simulink model "vipldws_fixpt"  (R2015b)
settings: Solver=FixedStepDiscrete  StartTime=0.0  StopTime=inf  RelTol=1e-3
model workspace (MATLAB code in the model file):
  | % Image size
  | imgSize = [240 360];
  | 
  | % Number of rows and columns in the image region to process.
  | numRows = floor(imgSize(1)/2);
  | numCols = imgSize(2);
  | 
  | % To handle different video sizes other than [240 360], scaling the Hough
  | % transform rho values by the below factor is required.
  | factor = sqrt(sum(imgSize.^2)) / sqrt(sum([240 360].^2));
  | 
  | %% parameters for the second lane
  | %approximately 35:45 (0-based index: 414:424)
  | startIdxRho_R = floor(factor * 414);
  | NumRhos_R = floor(factor * 11);
  | 
  | %approximately -90:-70 degrees (0-based index: 0:20)
  | startIdxTheta_R = 0;
  | NumThetas_R = 21;
  | neighborhood_R =  [min(7,NumRhos_R), min(7,NumThetas_R)];
  | 
  | %approximately 379:415 (0-based index: 0:35)
  | startIdxRho_L = floor(factor * 379);
  | NumRhos_L = floor(factor * 36);
  | 
  | %approximately 55:85 degrees (0-based index: 145: 175)
  | startIdxTheta_L = 145;
  | NumThetas_L = 21;
  | neighborhood_L =  [min(7,NumRhos_L), min(7,NumThetas_L)];
  | 
  | % Maximum number of lanes to find in the current frame.
  | expLaneNum = 2;
  | 
  | % Maximum number of lanes to store in the tracking repository.
  | maxLaneNum = 20;
  | 
  | % Angular resolution of Hough transform, i.e., the width of a theta bin is
  | % pi/angleNum.
  | angleNum = 180;
  | 
  | % Maximum allowable change of lane distance metric between two frames.
  | trackThreshold = 75;
  | 
  | % Minimum number of frames a lane must be detected to become a valid lane.
  | frameFound = 5;
  | 
  | % Maximum number of frames a lane can be missed without marking it invalid.
  | frameLost = 20;
  | 
  | % Size of the neighborhood around the maxima over which the Hough
  | % transforms values are suppressed. (Used in Find Local Maxima block)
  | neighborhood = [301, 81];
  | 
  | % Distance threshold for lane crossing warning; valid range is (0, 0.5).
  | thrWarn = 0.4;
  | 
  | % Weight (tweaking factor) of the angular difference for calculating the
  | % distance metric between two lanes. It is typically chosen to be close
  | % to the input image rows.
  | distanceMetricWeight = 200;
  | 
  | % Audio track used for lane cross warning.
  | load viprumbling.mat;
values from neighbouring files (symbols this model uses):
  param = getDefaultParameters()    [kalmanFilterForTracking.m]
undefined symbols (not defined in the file or in its folder): gray, High, len_measure, len_state, num_cols, num_rows, num_targets, Rec, SDTV, slselsubs
libraries: simulink x23, visiontextngfix x6, dspmtrx3 x5, visiontransforms x4, visionconversions x3, visionstatistics x3, dspindex x2, dspswit3 x2, dspsolvers x2, dspstat3 x2, dspquant2 x1, dspsigops x1
(part 2 of 3)

== system vipldws_fixpt/Departure Warning/Departure detection/check validity: right ==
  note: r1
      | r2
      | c1
      | c2
  note: r1
  note: r2
  note: c1
  note: c2
  note: valid lane [r1 c1 r2 c2]' if:
      | (1) r1 >= 0 [line outside image: e.g. [-1000 -1000 -1000 -1000]]
      | (2) r1~=r2 or c1 ~= c2 [point-not a line]
      | (3) abs(r1-c1)+abs(r2-c2) >=10 [noise]
      | (4) abs(c1-c2)<width-10 [almost horizontal line]
  In : Inport
  Abs2 : Abs
  Abs3 : Abs
  Add3 : Sum  Inputs=+-
  Add4 : Sum  Inputs=+-
  Add5 : Sum
  Compare To Constant1 : simulink/Logic and Bit Operations/Compare To Constant  relop=<  const=numCols-10  OutDataTypeStr=boolean  ZeroCross=off
  Compare To Constant2 : simulink/Logic and Bit Operations/Compare To Constant  relop=>=  const=10  OutDataTypeStr=boolean  ZeroCross=off
  Compare To Constant3 : simulink/Logic and Bit Operations/Compare To Constant  relop=>=  const=0  OutDataTypeStr=boolean  ZeroCross=off
  Logical Operator1 : Logic  Operator=OR  AllPortsSameDT=off  OutDataTypeStr=boolean
  Logical Operator7 : Logic  Inputs=4  AllPortsSameDT=off  OutDataTypeStr=boolean
  Multiport Selector2 : dspindex/Multiport Selector  rowsOrCols=Rows  idxCellArray={1,3,2,4}  idxErrMode=Generate Error
  Relational Operator2 : RelationalOperator  Operator=~=  OutDataTypeStr=boolean
  Relational Operator3 : RelationalOperator  Operator=~=  OutDataTypeStr=boolean
  Out : Outport
  wires:
  Logical Operator7/1 -> Out/1
  Compare To Constant2/1 -> Logical Operator7/3
  Logical Operator1/1 -> Logical Operator7/2
  Compare To Constant3/1 -> Logical Operator7/1
  In/1 -> Multiport Selector2/1
  Multiport Selector2/1 -> Relational Operator2/1, Compare To Constant3/1, Add3/1
  Multiport Selector2/3 -> Relational Operator3/1, Add4/1
  Multiport Selector2/4 -> Relational Operator3/2, Add4/2
  Relational Operator2/1 -> Logical Operator1/1
  Relational Operator3/1 -> Logical Operator1/2
  Add4/1 -> Abs3/1
  Add3/1 -> Abs2/1
  Abs2/1 -> Add5/1
  Abs3/1 -> Add5/2, Compare To Constant1/1
  Add5/1 -> Compare To Constant2/1
  Multiport Selector2/2 -> Relational Operator2/2, Add3/2
  Compare To Constant1/1 -> Logical Operator7/4

== system vipldws_fixpt/Departure Warning/Departure detection/subsystem ==
  note: Meaning of the message: 0 = Right lane departure, 1 = Normal driving, 2 = Left lane departure
  note: Normal Driving
  inMsg : Inport
  Combine Left Right Departure : MATLAB Function  TreatAsAtomicUnit=on
  Compare To Constant : simulink/Logic and Bit Operations/Compare To Constant  relop===  const=1  OutDataTypeStr=boolean  ZeroCross=off
  Compare To Constant1 : simulink/Logic and Bit Operations/Compare To Constant  relop=~=  const=1  OutDataTypeStr=boolean  ZeroCross=off
  Counter : dspswit3/Counter  Direction=Up  CountEvent=Non-zero sample  CounterSize=16 bits  MaxCount=255  InitialCount=0  Output=Count  HitValue=32  ResetInput=on  SamplesPerFrame=1  Ts=1  CntDtype=int32  HitDtype=Logical
  Delay : Delay  DelayLength=1  InitialCondition=int8(-1)  UseCircularBuffer=on
  Delay1 : Delay  DelayLength=1  InitialCondition=int8(-1)  UseCircularBuffer=on
  outMsg : Outport
  wires:
  Delay1/1 -> Compare To Constant1/1
  Combine Left Right Departure/1(outMsg) -> outMsg/1, Delay/1
  Counter/1 -> Combine Left Right Departure/3(numNormalDrivenFrames)
  Compare To Constant1/1 -> Counter/2
  Compare To Constant/1 -> Counter/1
  Delay/1 -> Combine Left Right Departure/2(prevMsg)
  inMsg/1 -> Compare To Constant/1, Delay1/1, Combine Left Right Departure/1(curMsg)

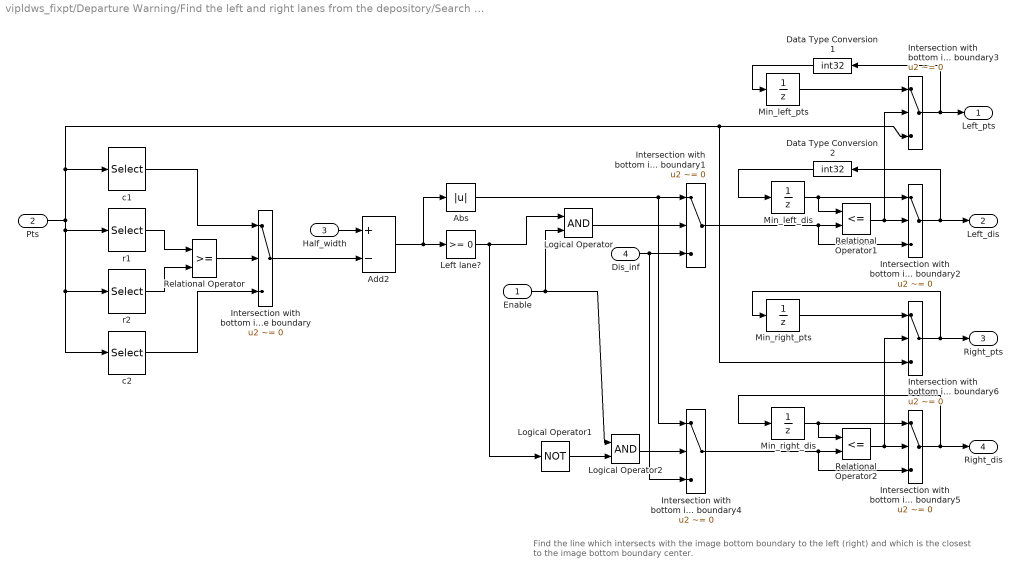
== system vipldws_fixpt/Departure Warning/Find the left and right lanes from the depository/Search for the left and right lanes ==
  note: Find the line which intersects with the image bottom boundary to the left (right) and which is the closest to the image bottom boundary center.
  Enable : Inport
  Pts : Inport  Port=2
  Half_width : Inport  Port=3
  Dis_inf : Inport  Port=4
  Abs : Abs
  Add2 : Sum  Inputs=+-
  Data Type Conversion1 : DataTypeConversion  OutDataTypeStr=int32  SaturateOnIntegerOverflow=on  RndMeth=Zero
  Data Type Conversion2 : DataTypeConversion  OutDataTypeStr=int32  SaturateOnIntegerOverflow=on  RndMeth=Zero
  Intersection with bottom image boundary{,1..6} (7 alike) : Switch  Criteria=u2 ~= 0  ZeroCross=off
  Left lane? : simulink/Logic and Bit Operations/Compare To Zero  relop=>=  OutDataTypeStr=boolean  ZeroCross=off
  Logical Operator : Logic  AllPortsSameDT=off  OutDataTypeStr=boolean
  Logical Operator1 : Logic  Operator=NOT  AllPortsSameDT=off  OutDataTypeStr=boolean
  Logical Operator2 : Logic  AllPortsSameDT=off  OutDataTypeStr=boolean
  Min_left_dis : UnitDelay  InitialCondition=single(intmax('int16'))  SampleTime=-1
  Min_left_pts : UnitDelay  InitialCondition=[0; 0; 0; 0]  SampleTime=-1
  Min_right_dis : UnitDelay  InitialCondition=single(intmax('int16'))  SampleTime=-1
  Min_right_pts : UnitDelay  InitialCondition=[0; 0; 0; 0]  SampleTime=-1
  Relational Operator : RelationalOperator  OutDataTypeStr=boolean  ZeroCross=off
  Relational Operator1 : RelationalOperator  Operator=<=  OutDataTypeStr=boolean
  Relational Operator2 : RelationalOperator  Operator=<=  OutDataTypeStr=boolean
  c1 : Selector  InputPortWidth=4  IndexOptions=Index vector (dialog)  Indices=2  OutputSizes=1
  c2 : Selector  InputPortWidth=4  IndexOptions=Index vector (dialog)  Indices=4  OutputSizes=1
  r1 : Selector  InputPortWidth=4  IndexOptions=Index vector (dialog)  Indices=1  OutputSizes=1
  r2 : Selector  InputPortWidth=4  IndexOptions=Index vector (dialog)  Indices=3  OutputSizes=1
  Left_pts : Outport
  Left_dis : Outport  Port=2
  Right_pts : Outport  Port=3
  Right_dis : Outport  Port=4
  wires:
  Logical Operator1/1 -> Logical Operator2/2
  Logical Operator2/1 -> Intersection with bottom image boundary4/2
  Enable/1 -> Logical Operator2/1, Logical Operator/2
  Left lane?/1 -> Logical Operator1/1, Logical Operator/1
  Logical Operator/1 -> Intersection with bottom image boundary1/2
  Half_width/1 -> Add2/1
  Intersection with bottom image boundary6/1 -> Min_right_pts/1, Right_pts/1
  Min_right_pts/1 -> Intersection with bottom image boundary6/1
  Intersection with bottom image boundary5/1 -> Right_dis/1, Min_right_dis/1
  Intersection with bottom image boundary4/1 -> Relational Operator2/2, Intersection with bottom image boundary5/3
  Relational Operator2/1 -> Intersection with bottom image boundary5/2, Intersection with bottom image boundary6/2
  Min_right_dis/1 -> Intersection with bottom image boundary5/1, Relational Operator2/1
  Pts/1 -> Intersection with bottom image boundary3/3, Intersection with bottom image boundary6/3, c1/1, r1/1, c2/1, r2/1
  Intersection with bottom image boundary3/1 -> Left_pts/1, Data Type Conversion1/1
  Min_left_pts/1 -> Intersection with bottom image boundary3/1
  Intersection with bottom image boundary2/1 -> Left_dis/1, Data Type Conversion2/1
  Intersection with bottom image boundary1/1 -> Intersection with bottom image boundary2/3, Relational Operator1/2
  Dis_inf/1 -> Intersection with bottom image boundary4/3, Intersection with bottom image boundary1/3
  Abs/1 -> Intersection with bottom image boundary4/1, Intersection with bottom image boundary1/1
  Relational Operator1/1 -> Intersection with bottom image boundary3/2, Intersection with bottom image boundary2/2
  Min_left_dis/1 -> Relational Operator1/1, Intersection with bottom image boundary2/1
  Add2/1 -> Abs/1, Left lane?/1
  Intersection with bottom image boundary/1 -> Add2/2
  c2/1 -> Intersection with bottom image boundary/3
  c1/1 -> Intersection with bottom image boundary/1
  Relational Operator/1 -> Intersection with bottom image boundary/2
  r2/1 -> Relational Operator/2
  r1/1 -> Relational Operator/1
  Data Type Conversion1/1 -> Min_left_pts/1
  Data Type Conversion2/1 -> Min_left_dis/1

== system vipldws_fixpt/Lane Detection/Peak detection/Enable signal generator ==
  Num : Inport
  Assignment : Assignment  NumberOfDimensions=2  IndexOptions=Assign all,Index vector (port)  Indices=-1,1  OutputSizes=1,1
  Constant : Constant  Value=zeros(1, expLaneNum)  VectorParams1D=off  OutDataTypeStr=boolean
  Constant1 : Constant  VectorParams1D=off  OutDataTypeStr=boolean
  For Iterator : ForIterator  ResetStates=reset  IterationSource=external
  Enable : Outport
  wires:
  For Iterator/1 -> Assignment/3
  Constant1/1 -> Assignment/2
  Assignment/1 -> Enable/1
  Constant/1 -> Assignment/1
  Num/1 -> For Iterator/1

== system vipldws_fixpt/Lane Tracking/Kalman Filter (In order to change fixed-point data settings, the link to the library is disabled.)/Control ==
  Z : Inport
  Enable : Inport  Port=2
  En_delay : Inport  Port=3
  X : Inport  Port=4
  P : Inport  Port=5
  En_Not : Logic  Operator=NOT  AllPortsSameDT=off
  En_Or : Logic  Operator=OR  AllPortsSameDT=off
  En_Selector : Selector  NumberOfDimensions=2  IndexOptions=Select all,Index vector (port)  Indices=-1,1  OutputSizes=1
  Iterator : ForIterator  IterationLimit=num_targets
  Options : Subsystem
  Rst_And : Logic  AllPortsSameDT=off
  Rst_Selector : Selector  NumberOfDimensions=2  IndexOptions=Select all,Index vector (port)  Indices=-1,1  OutputSizes=1
  Z_est : Outport
  Z_prd : Outport  Port=2
  X_prd : Outport  Port=3
  P_prd : Outport  Port=4
  wires:
  Options/2(Z_prd) -> Z_prd/1
  Iterator/1 -> Options/3(Index), En_Selector/2, Rst_Selector/2
  Options/1(Z_est) -> Z_est/1
  Options/3(X_prd) -> X_prd/1
  Options/4(P_prd) -> P_prd/1
  Z/1 -> Options/4(Z)
  X/1 -> Options/5(X)
  P/1 -> Options/6(P)
  Enable/1 -> En_Selector/1
  En_delay/1 -> Rst_Selector/1
  En_Selector/1 -> En_Not/1, En_Or/1, Options/1(En_core)
  En_Not/1 -> Rst_And/1
  Rst_Selector/1 -> Rst_And/2
  Rst_And/1 -> En_Or/2, Options/2(Reset)
  En_Or/1 -> Options/Enable

== system vipldws_fixpt/Lane Tracking/Matching/Calculate the distances between the lines found in the current frame and those in the repository ==
  Count : Inport
  Rep_ref : Inport  Port=2
  Line : Inport  Port=3
  Enable : Inport  Port=4
  For Iterator : ForIterator  ResetStates=reset  IterationLimit=maxLaneNum
  "Select a line from the repository; if it is valid (Count > 0), Calculate its distance to the input lines." : Subsystem
  Selector1 : Selector  NumberOfDimensions=2  InputPortWidth=3  IndexOptions=Select all,Index vector (port)  Indices=-1,-1  OutputSizes=1
  Dis : Outport
  wires:
  Selector1/1 -> "Select a line from the repository; if it is valid (Count > 0), Calculate its distance to the input lines."/Enable
  Count/1 -> Selector1/1
  Line/1 -> "Select a line from the repository; if it is valid (Count > 0), Calculate its distance to the input lines."/3(Line)
  Rep_ref/1 -> "Select a line from the repository; if it is valid (Count > 0), Calculate its distance to the input lines."/2(Rep_ref)
  "Select a line from the repository; if it is valid (Count > 0), Calculate its distance to the input lines."/1(Dis) -> Dis/1
  For Iterator/1 -> "Select a line from the repository; if it is valid (Count > 0), Calculate its distance to the input lines."/1(Idx), Selector1/2
  Enable/1 -> "Select a line from the repository; if it is valid (Count > 0), Calculate its distance to the input lines."/4(Enable)

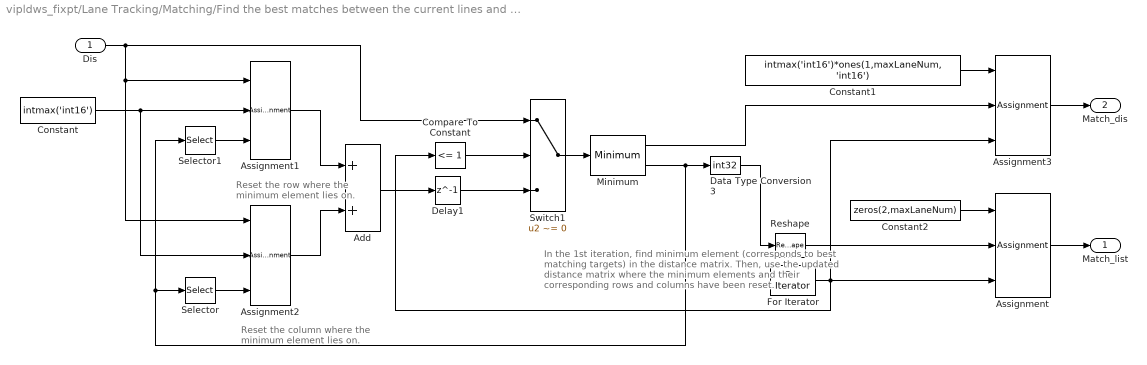
== system vipldws_fixpt/Lane Tracking/Matching/Find the best matches between the current lines and those in the repository ==
  note: Reset the row where the
      | minimum element lies on.
  note: Reset the column where the
      | minimum element lies on.
  note: In the 1st iteration, find minimum element (corresponds to
      | best matching targets) in the distance matrix. Then, use the
      | updated distance matrix where the minimum elements and
      | their  corresponding rows and columns have been reset.
  Dis : Inport
  Add : Sum
  Assignment : Assignment  NumberOfDimensions=2  IndexOptions=Assign all,Index vector (port)  Indices=-1,-1  OutputSizes=1,1
  Assignment1 : Assignment  NumberOfDimensions=2  IndexOptions=Index vector (port),Assign all  Indices=1,-1  OutputSizes=1,1
  Assignment2 : Assignment  NumberOfDimensions=2  IndexOptions=Assign all,Index vector (port)  Indices=-1,-1  OutputSizes=1,1
  Assignment3 : Assignment  NumberOfDimensions=2  IndexOptions=Assign all,Index vector (port)  Indices=-1,-1  OutputSizes=1,1
  Compare To Constant : simulink/Logic and Bit Operations/Compare To Constant  relop=<=  const=1  OutDataTypeStr=boolean  ZeroCross=off
  Constant : Constant  Value=intmax('int16')  VectorParams1D=off  OutDataTypeStr=Inherit: Inherit via back propagation
  Constant1 : Constant  Value=intmax('int16')*ones(1,maxLaneNum, 'int16')  VectorParams1D=off  OutDataTypeStr=Inherit: Inherit via back propagation
  Constant2 : Constant  Value=zeros(2,maxLaneNum)  VectorParams1D=off  OutDataTypeStr=Inherit: Inherit via back propagation
  Data Type Conversion3 : DataTypeConversion  OutDataTypeStr=int32  SaturateOnIntegerOverflow=on  RndMeth=Zero
  Delay1 : Delay  DelayLength=1  InitialCondition=0  UseCircularBuffer=on
  For Iterator : ForIterator  IterationLimit=expLaneNum
  Minimum : dspstat3/Minimum  fcn=Value and Index  reset=None  InputProcessing=Columns as channels (frame based)  indexBase=One  operateOver=Entire input  Dimension=1  operation=minimum  roiEnable=off  roiType=Rectangles  roiPortion=Entire ROI  roiOutput=Individual statistics for each ROI  roiFlag=off  roundingMode=Floor  overflowMode=off
  Reshape : Reshape  OutputDimensionality=Column vector (2-D)
  Selector : Selector  InputPortWidth=2  IndexOptions=Index vector (dialog)  Indices=[2]  OutputSizes=1
  Selector1 : Selector  InputPortWidth=2  IndexOptions=Index vector (dialog)  Indices=[1]  OutputSizes=1
  Switch1 : Switch  Criteria=u2 ~= 0
  Match_list : Outport
  Match_dis : Outport  Port=2
  wires:
  Reshape/1 -> Assignment/2
  Constant/1 -> Assignment2/2, Assignment1/2
  Minimum/1 -> Assignment3/2
  Minimum/2 -> Selector1/1, Selector/1, Data Type Conversion3/1
  Assignment3/1 -> Match_dis/1
  Add/1 -> Delay1/1
  Assignment2/1 -> Add/2
  Assignment1/1 -> Add/1
  Selector1/1 -> Assignment1/3
  Selector/1 -> Assignment2/3
  Assignment/1 -> Match_list/1
  Delay1/1 -> Switch1/3
  Dis/1 -> Switch1/1, Assignment1/1, Assignment2/1
  Switch1/1 -> Minimum/1
  For Iterator/1 -> Assignment3/3, Assignment/3, Compare To Constant/1
  Compare To Constant/1 -> Switch1/2
  Data Type Conversion3/1 -> Reshape/1
  Constant1/1 -> Assignment3/1
  Constant2/1 -> Assignment/1

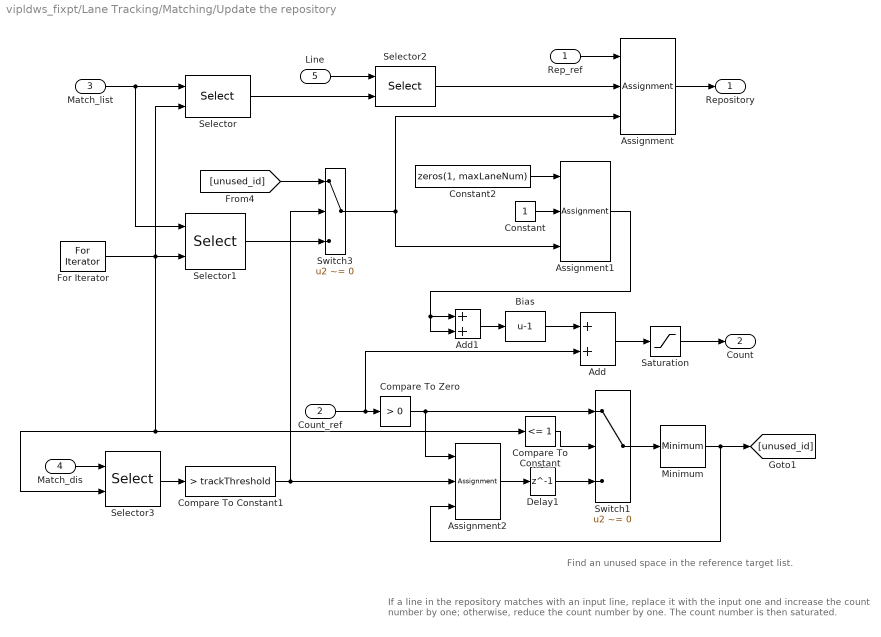
== system vipldws_fixpt/Lane Tracking/Matching/Update the repository ==
  note: If a line in the repository matches with an input line, replace it with the input one and increase the count number by one;
      | otherwise, reduce the count number by one. The count number is then saturated.
  note: Find an unused space in the reference target list.
  Rep_ref : Inport
  Count_ref : Inport  Port=2
  Match_list : Inport  Port=3
  Match_dis : Inport  Port=4
  Line : Inport  Port=5
  Add : Sum  InputSameDT=on
  Add1 : Sum  OutDataTypeStr=int32  InputSameDT=on
  Assignment : Assignment  NumberOfDimensions=2  IndexOptions=Assign all,Starting index (port)  Indices=-1,-1  OutputSizes=1,1
  Assignment1 : Assignment  NumberOfDimensions=2  IndexOptions=Assign all,Index vector (port)  Indices=-1,-1  OutputSizes=slselsubs([1, num_targets],1),slselsubs([1, num_targets],2)
  Assignment2 : Assignment  IndexOptions=Index vector (port)  Indices=-1  OutputSizes=[1, num_targets]
  Bias : Bias  Bias=-1
  Compare To Constant : simulink/Logic and Bit Operations/Compare To Constant  relop=<=  const=1  OutDataTypeStr=boolean  ZeroCross=off
  Compare To Constant1 : simulink/Logic and Bit Operations/Compare To Constant  relop=>  const=trackThreshold  OutDataTypeStr=boolean  ZeroCross=off
  Compare To Zero : simulink/Logic and Bit Operations/Compare To Zero  relop=>  OutDataTypeStr=boolean  ZeroCross=off
  Constant : Constant  VectorParams1D=off  OutDataTypeStr=Inherit: Inherit via back propagation
  Constant2 : Constant  Value=zeros(1, maxLaneNum)  VectorParams1D=off  OutDataTypeStr=int32
  Delay1 : Delay  DelayLength=1  InitialCondition=0  UseCircularBuffer=on
  For Iterator : ForIterator  ResetStates=reset  IterationLimit=expLaneNum
  Minimum : dspstat3/Minimum  fcn=Index  reset=None  InputProcessing=Columns as channels (frame based)  indexBase=One  operateOver=Each row  Dimension=1  operation=minimum  roiEnable=off  roiType=Rectangles  roiPortion=Entire ROI  roiOutput=Individual statistics for each ROI  roiFlag=off  roundingMode=Floor  overflowMode=off
  Saturation : Saturate  UpperLimit=frameFound+frameLost  LowerLimit=0
  Selector : Selector  NumberOfDimensions=2  InputPortWidth=3  IndexOptions=Index vector (dialog),Index vector (port)  Indices=[2],[1]  OutputSizes=1
  Selector1 : Selector  NumberOfDimensions=2  InputPortWidth=3  IndexOptions=Index vector (dialog),Index vector (port)  Indices=[1],[2]  OutputSizes=1
  Selector2 : Selector  NumberOfDimensions=2  InputPortWidth=3  IndexOptions=Select all,Index vector (port)  Indices=-1,1  OutputSizes=1
  Selector3 : Selector  NumberOfDimensions=2  InputPortWidth=3  IndexOptions=Select all,Index vector (port)  Indices=-1,-1  OutputSizes=1
  Switch1 : Switch  Criteria=u2 ~= 0
  Switch3 : Switch  Criteria=u2 ~= 0
  Repository : Outport
  Count : Outport  Port=2
  wires:
  Saturation/1 -> Count/1
  Selector3/1 -> Compare To Constant1/1
  Rep_ref/1 -> Assignment/1
  Compare To Zero/1 -> Assignment2/1, Switch1/1
  Add/1 -> Saturation/1
  Bias/1 -> Add/1
  Add1/1 -> Bias/1
  Selector2/1 -> Assignment/2
  For Iterator/1 -> Selector1/2, Selector/2, Compare To Constant/1, Selector3/2
  Compare To Constant/1 -> Switch1/2
  Match_list/1 -> Selector1/1, Selector/1
  Line/1 -> Selector2/1
  Assignment/1 -> Repository/1
  Assignment1/1 -> Add1/2, Add1/1
  Match_dis/1 -> Selector3/1
  Assignment2/1 -> Delay1/1
  Minimum/1 -> Assignment2/3, [unused_id]
  Switch1/1 -> Minimum/1
  Count_ref/1 -> Compare To Zero/1, Add/2
  Delay1/1 -> Switch1/3
  Compare To Constant1/1 -> Assignment2/2, Switch3/2
  [unused_id] -> Switch3/1
  Selector/1 -> Selector2/2
  Selector1/1 -> Switch3/3
  Switch3/1 -> Assignment/3, Assignment1/3
  Constant/1 -> Assignment1/2
  Constant2/1 -> Assignment1/1

== system vipldws_fixpt/Output/Subsystem/Draw  Polygon ==
  inPts : Inport
  RGB : Inport  Port=2
  Enable : EnablePort  PropagateVarSize=During execution
  DrawShapes : visiontextngfix/Draw Shapes  shape=Polygons  fill=on  lineWidth=1  fillClrSource=Specify via dialog  display=User-specified value  intensity=200  color=255 * [0 1 1]  opacity=0.2  viewport=Entire image  antialiasing=off  inType=Obsolete  imagePorts=One multidimensional signal  prodOutputMode=Binary point scaling  prodOutputWordLength=32  prodOutputFracLength=14  memoryMode=Specify word length  memoryWordLength=16  memoryFracLength=15  roundingMode=Floor  overflowMode=off
  Line to Polygon Coordinates : Subsystem
  Selector2 : Selector  NumberOfDimensions=2  InputPortWidth=3  IndexOptions=Index vector (dialog),Select all  Indices=[2 1 4 3 6 5 8 7 10 9 12 11],1  OutputSizes=1,1
  Transpose1 : Math  Operator=transpose  SaturateOnIntegerOverflow=on
  RGBout : Outport
  wires:
  inPts/1 -> Line to Polygon Coordinates/1(Pts_line)
  DrawShapes/1 -> RGBout/1
  RGB/1 -> DrawShapes/1
  Selector2/1 -> Transpose1/1
  Line to Polygon Coordinates/1(Pts_polygon) -> Selector2/1
  Transpose1/1 -> DrawShapes/2

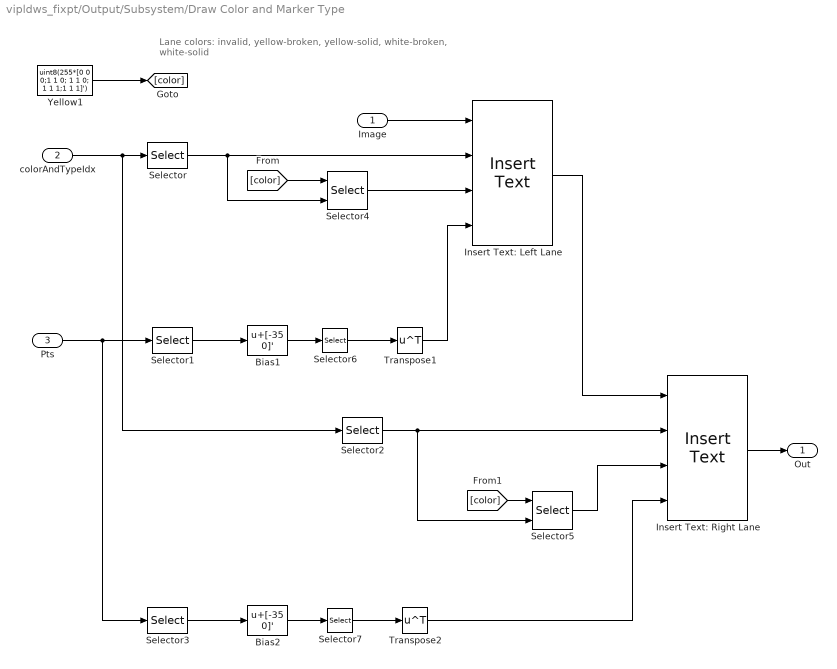
== system vipldws_fixpt/Output/Subsystem/Draw Color and Marker Type ==
  note: Lane colors:
      | invalid, yellow-broken, yellow-solid, white-broken, white-solid
  Image : Inport
  colorAndTypeIdx : Inport  Port=2
  Pts : Inport  Port=3
  Bias1 : Bias  Bias=[-35 0]'
  Bias2 : Bias  Bias=[-35 0]'
  Insert Text: Left Lane : visiontextngfix/Insert Text  inputType=Obsolete  theText={'',sprintf('Yellow\nBroken'),sprintf('Yellow\nSolid'),sprintf('White\nBroken'),sprintf('White\nSolid')}  getTextLocFrom=Input port  textLoc=[170 2]  getTextColorFrom=Input port  textColor=[1 1 1]  getTextIntensityFrom=Specify via dialog  textIntensity=0  getTextOpacityFrom=Specify via dialog  textOpacity=1  dummyVar2=0  dummyVar3=0  dummyVar4=0  imagePorts=One multidimensional signal  isInputTransposed=off  fontFace=LucidaTypewriterBold  dummyVar1=0  blockFontSize=14  antiAliased=on
  Insert Text: Right Lane : visiontextngfix/Insert Text  inputType=Obsolete  theText={'',sprintf('Yellow\nBroken'),sprintf('Yellow\nSolid'),sprintf('White\nBroken'),sprintf('White\nSolid')}  getTextLocFrom=Input port  textLoc=[170 2]  getTextColorFrom=Input port  textColor=[1 1 1]  getTextIntensityFrom=Specify via dialog  textIntensity=0  getTextOpacityFrom=Specify via dialog  textOpacity=1  dummyVar2=0  dummyVar3=0  dummyVar4=0  imagePorts=One multidimensional signal  isInputTransposed=off  fontFace=LucidaTypewriterBold  dummyVar1=0  blockFontSize=14  antiAliased=on
  Selector : Selector  IndexMode=Zero-based  InputPortWidth=2  IndexOptions=Index vector (dialog)  Indices=0  OutputSizes=1
  Selector1 : Selector  NumberOfDimensions=2  IndexMode=Zero-based  InputPortWidth=2  IndexOptions=Index vector (dialog),Index vector (dialog)  Indices=0:1,0  OutputSizes=1,1
  Selector2 : Selector  IndexMode=Zero-based  InputPortWidth=2  IndexOptions=Index vector (dialog)  Indices=1  OutputSizes=1
  Selector3 : Selector  NumberOfDimensions=2  IndexMode=Zero-based  InputPortWidth=2  IndexOptions=Index vector (dialog),Index vector (dialog)  Indices=0:1,1  OutputSizes=1,1
  Selector4 : Selector  NumberOfDimensions=2  InputPortWidth=3  IndexOptions=Select all,Index vector (port)  Indices=[1 3],1  OutputSizes=1,1
  Selector5 : Selector  NumberOfDimensions=2  InputPortWidth=3  IndexOptions=Select all,Index vector (port)  Indices=[1 3],1  OutputSizes=1,1
  Selector6 : Selector  NumberOfDimensions=2  InputPortWidth=3  IndexOptions=Index vector (dialog),Select all  Indices=[2 1],[2 1]  OutputSizes=1,1
  Selector7 : Selector  NumberOfDimensions=2  InputPortWidth=3  IndexOptions=Index vector (dialog),Select all  Indices=[2 1],1  OutputSizes=1,1
  Transpose1 : Math  Operator=transpose  SaturateOnIntegerOverflow=on
  Transpose2 : Math  Operator=transpose  SaturateOnIntegerOverflow=on
  Yellow1 : Constant  Value="uint8(255*[0 0  0;1 1 0; 1 1 0; 1 1 1;1 1 1]')"  VectorParams1D=off  OutDataTypeStr=uint8
  Out : Outport
  wires:
  Selector4/1 -> Insert Text: Left Lane/3
  Selector/1 -> Insert Text: Left Lane/2, Selector4/2
  Selector1/1 -> Bias1/1
  Image/1 -> Insert Text: Left Lane/1
  colorAndTypeIdx/1 -> Selector/1, Selector2/1
  Insert Text: Left Lane/1 -> Insert Text: Right Lane/1
  Pts/1 -> Selector1/1, Selector3/1
  Selector5/1 -> Insert Text: Right Lane/3
  Selector2/1 -> Insert Text: Right Lane/2, Selector5/2
  Selector3/1 -> Bias2/1
  Insert Text: Right Lane/1 -> Out/1
  [color] -> Selector4/1
  [color] -> Selector5/1
  Yellow1/1 -> [color]
  Selector6/1 -> Transpose1/1
  Bias1/1 -> Selector6/1
  Transpose1/1 -> Insert Text: Left Lane/4
  Selector7/1 -> Transpose2/1
  Bias2/1 -> Selector7/1
  Transpose2/1 -> Insert Text: Right Lane/4

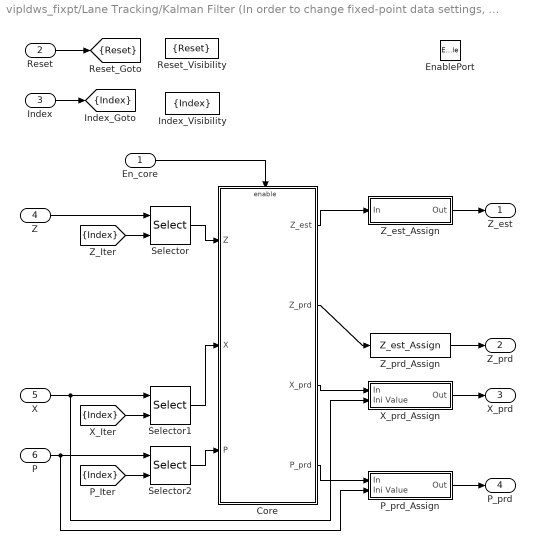
== system vipldws_fixpt/Lane Tracking/Kalman Filter (In order to change fixed-point data settings, the link to the library is disabled.)/Control/Options ==
  En_core : Inport
  Reset : Inport  Port=2
  Index : Inport  Port=3
  Z : Inport  Port=4
  X : Inport  Port=5
  P : Inport  Port=6
  EnablePort : EnablePort  PropagateVarSize=During execution
  Core : Subsystem
  Index_Visibility : GotoTagVisibility  GotoTag=Index
  P_prd_Assign : Subsystem
  Reset_Visibility : GotoTagVisibility  GotoTag=Reset
  Selector : Selector  NumberOfDimensions=2  InputPortWidth=3  IndexOptions=Select all,Index vector (port)  Indices=-1,1  OutputSizes=1
  Selector1 : Selector  NumberOfDimensions=2  InputPortWidth=3  IndexOptions=Select all,Index vector (port)  Indices=-1,1  OutputSizes=1
  Selector2 : Selector  NumberOfDimensions=2  InputPortWidth=3  IndexOptions=Select all,Index vector (port)  Indices=-1,1  OutputSizes=1
  X_prd_Assign : Subsystem
  Z_est_Assign : Subsystem  mask{reset_value=zeros(len_measure, 1), num_rows=len_measure, num_cols=num_targets}
      mask prompts: reset_value "Default values:"; num_rows "Number of rows:"; num_cols "Number of Columns:"
      mask Display: disp('Assign/reset')
  Z_prd_Assign : dspadpt3/Kalman Filter/Control/Options/Z_est_Assign  reset_value=zeros(len_measure, 1)  num_rows=len_measure  num_cols=num_targets
  Z_est : Outport
  Z_prd : Outport  Port=2
  X_prd : Outport  Port=3
  P_prd : Outport  Port=4
  tag scope: Index=scoped, Reset=scoped
  wires:
  Z_prd_Assign/1 -> Z_prd/1
  Core/2(Z_prd) -> Z_prd_Assign/1
  Selector/1 -> Core/1(Z)
  X/1 -> Selector1/1, X_prd_Assign/2(Ini Value)
  [Index] -> Selector/2
  [Index] -> Selector2/2
  [Index] -> Selector1/2
  P/1 -> Selector2/1, P_prd_Assign/2(Ini Value)
  Z/1 -> Selector/1
  Selector1/1 -> Core/2(X)
  Selector2/1 -> Core/3(P)
  Core/3(X_prd) -> X_prd_Assign/1(In)
  X_prd_Assign/1(Out) -> X_prd/1
  Core/1(Z_est) -> Z_est_Assign/1(In)
  Core/4(P_prd) -> P_prd_Assign/1(In)
  Z_est_Assign/1(Out) -> Z_est/1
  P_prd_Assign/1(Out) -> P_prd/1
  Index/1 -> [Index]
  Reset/1 -> [Reset]
  En_core/1 -> Core/Enable

== system vipldws_fixpt/Lane Tracking/Matching/Calculate the distances between the lines found in the current frame and those in the repository/Select a line from the repository; if it is valid (Count > 0), Calculate its distance to the input lines. ==
  Idx : Inport
  Rep_ref : Inport  Port=2
  Line : Inport  Port=3
  Enable : Inport  Port=4
  EnablePort : EnablePort  StatesWhenEnabling=reset  PropagateVarSize=During execution
  Assignment : Assignment  NumberOfDimensions=2  IndexOptions=Index vector (port),Assign all  Indices=-1,-1  OutputSizes=1,1
  Calculate the distances between the chosen line in the repository and all input lines. : Subsystem  TreatAsAtomicUnit=on
  Constant2 : Constant  Value=intmax('int16') * ones(maxLaneNum,'int16')  VectorParams1D=off  OutDataTypeStr=int32
  Selector1 : Selector  NumberOfDimensions=2  InputPortWidth=3  IndexOptions=Index vector (port),Select all  Indices=-1,-1  OutputSizes=1
  Selector2 : Selector  NumberOfDimensions=2  InputPortWidth=3  IndexOptions=Select all,Index vector (port)  Indices=-1,-1  OutputSizes=1
  Dis : Outport
  wires:
  Constant2/1 -> Assignment/1, Selector1/1
  Calculate the distances between the chosen line in the repository and all input lines./1(Dis_out) -> Assignment/2
  Assignment/1 -> Dis/1
  Idx/1 -> Selector1/2, Assignment/3, Selector2/2
  Selector1/1 -> Calculate the distances between the chosen line in the repository and all input lines./1(Dis)
  Line/1 -> Calculate the distances between the chosen line in the repository and all input lines./3(Line)
  Selector2/1 -> Calculate the distances between the chosen line in the repository and all input lines./2(Rep_ref)
  Enable/1 -> Calculate the distances between the chosen line in the repository and all input lines./4(Enable)
  Rep_ref/1 -> Selector2/1

== system vipldws_fixpt/Output/Subsystem/Draw  Polygon/Line to Polygon Coordinates ==
  note: R2    or    239
      | C2    or    359
  note: R2
      | C2
  note: r2     or   239
      | c2     or    0
  note: r2
      | c2
  note: r2
      | c2
  note: r1
      | c1
      | ----
      | r2
      | c2
      | ----
      | r2     or   239
      | c2     or    0
      | ------
      | R2    or    239
      | C2    or    359
      | -----
      | R2
      | C2
      | -----
      | R1
      | C1
  note: R2
      | C2
  note: (R1,C1)
      |  \
      |        \
      |            \
      |                  \
      |                        (R2,C2)
  note: (r1,c1)
      |                        /
      |                    /
      |               /
      |          /
      | (r2,c2)
  note: R1
      | C1
  note: r1
      | c1
  note: r1   R1
      | c1   C1
      | r2   R2
      | c2   C2
  Pts_line : Inport
  DSP Constant : Constant  Value=[239 0]'  VectorParams1D=off  OutDataTypeStr=int32  SampleTime=1/30
  DSP Constant2 : Constant  Value=[239 359]'  VectorParams1D=off  OutDataTypeStr=int32  SampleTime=1/30
  Matrix Concatenation6 : Concatenate  NumInputs=6  Mode=Multidimensional array
  Selector : Selector  NumberOfDimensions=2  InputPortWidth=3  IndexOptions=Index vector (dialog),Index vector (dialog)  Indices=3:4,2  OutputSizes=1
  Selector1 : Selector  NumberOfDimensions=2  InputPortWidth=3  IndexOptions=Index vector (dialog),Index vector (dialog)  Indices=1:2,1  OutputSizes=1
  Selector2 : Selector  NumberOfDimensions=2  InputPortWidth=3  IndexOptions=Index vector (dialog),Index vector (dialog)  Indices=1:2,2  OutputSizes=1
  Selector3 : Selector  InputPortWidth=2  IndexOptions=Index vector (dialog)  Indices=1  OutputSizes=1
  Selector4 : Selector  NumberOfDimensions=2  InputPortWidth=3  IndexOptions=Index vector (dialog),Index vector (dialog)  Indices=3:4,1  OutputSizes=1
  Selector5 : Selector  InputPortWidth=2  IndexOptions=Index vector (dialog)  Indices=1  OutputSizes=1
  Switch : Switch  Threshold=239
  Switch1 : Switch  Threshold=239
  Pts_polygon : Outport
  wires:
  Pts_line/1 -> Selector2/1, Selector/1, Selector4/1, Selector1/1
  Switch1/1 -> Matrix Concatenation6/4
  Switch/1 -> Matrix Concatenation6/3
  Selector2/1 -> Matrix Concatenation6/6
  DSP Constant2/1 -> Switch1/3
  Selector5/1 -> Switch1/2  "R2"
  DSP Constant/1 -> Switch/3
  Selector4/1 -> Matrix Concatenation6/2, Selector3/1, Switch/1
  Selector3/1 -> Switch/2  "r2"
  Matrix Concatenation6/1 -> Pts_polygon/1
  Selector/1 -> Matrix Concatenation6/5, Selector5/1, Switch1/1
  Selector1/1 -> Matrix Concatenation6/1

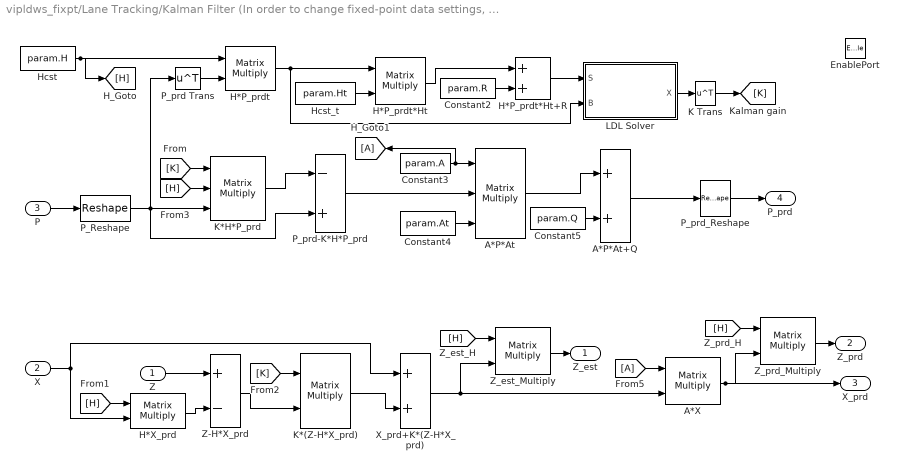
== system vipldws_fixpt/Lane Tracking/Kalman Filter (In order to change fixed-point data settings, the link to the library is disabled.)/Control/Options/Core ==
  Z : Inport
  X : Inport  Port=2
  P : Inport  Port=3
  EnablePort : EnablePort  PropagateVarSize=During execution
  A*P*At : Product  Inputs=3  Multiplication=Matrix(*)  InputSameDT=on  OutDataTypeStr=Inherit: Same as first input
  A*P*At+Q : Sum  InputSameDT=on  OutDataTypeStr=Inherit: Same as first input
  A*X : Product  Multiplication=Matrix(*)  InputSameDT=on  OutDataTypeStr=Inherit: Same as first input
  Constant2 : Constant  Value=param.R  VectorParams1D=off  OutDataTypeStr=Inherit: Inherit via back propagation
  Constant3 : Constant  Value=param.A  VectorParams1D=off  OutDataTypeStr=Inherit: Inherit via back propagation
  Constant4 : Constant  Value=param.At  VectorParams1D=off  OutDataTypeStr=Inherit: Inherit via back propagation
  Constant5 : Constant  Value=param.Q  VectorParams1D=off  OutDataTypeStr=Inherit: Inherit via back propagation
  H*P_prdt : Product  Multiplication=Matrix(*)  InputSameDT=on  OutDataTypeStr=Inherit: Same as first input
  H*P_prdt*Ht : Product  Multiplication=Matrix(*)  OutDataTypeStr=Inherit: Inherit via back propagation  InputSameDT=on
  H*P_prdt*Ht+R : Sum  OutDataTypeStr=Inherit: Inherit via back propagation  InputSameDT=on
  H*X_prd : Product  Multiplication=Matrix(*)  OutDataTypeStr=Inherit: Inherit via back propagation  InputSameDT=on
  Hcst : Constant  Value=param.H  VectorParams1D=off  OutDataTypeStr=Inherit: Inherit via back propagation
  Hcst_t : Constant  Value=param.Ht  VectorParams1D=off  OutDataTypeStr=Inherit: Inherit via back propagation
  K Trans : Math  Operator=transpose  SaturateOnIntegerOverflow=on
  K*(Z-H*X_prd) : Product  Multiplication=Matrix(*)  InputSameDT=on  OutDataTypeStr=Inherit: Same as first input
  K*H*P_prd : Product  Inputs=3  Multiplication=Matrix(*)  InputSameDT=on  OutDataTypeStr=Inherit: Same as first input
  LDL Solver : Subsystem  AncestorBlock=dspsolvers/LDL Solver  mask(LDL Solver){errmode=Warning}
      mask prompts: errmode "Non-positive definite input:"
      mask help: Solve SX=B using LDL' factorization. Only for use with a symmetric (Hermitian) positive definite input matrix S. S must be square. B must have the same number of rows as S.
      mask init:
      | Bcols=1;
      | x=[ 0.135 0.475 .475 0.135 0.135 NaN .135 .475 NaN 0.55 0.64 0.64 0.55 0.55 NaN 0.685 0.73 NaN 0.685 0.73 NaN 0.775 0.865 0.865 0.775 0.775 ];
      | y=[ 0.2 0.2 0.7 0.7 0.2 NaN .7 .2 NaN 0.2 0.2 0.7 0.7 0.2 NaN 0.4 0.4 NaN 0.45 0.45 NaN 0.2 0.2 0.7 0.7 0.2 ];
      | %
      | set_param([gcb '/LDL Factorization'],'errmode',get_param(gcb,'errmode'));
      settings: RTWMemSecFuncInitTerm=Default  RTWMemSecFuncExecute=Default  RTWMemSecDataConstants=Default  RTWMemSecDataInternal=Default  RTWMemSecDataParameters=Default
      mask Help: eval('blocksethelp');
      mask TypeOptions errmode: Ignore | Warning | Error
      mask Display:
      | plot(x,y+0.05);
      | text(0.17,0.9,'SX=B (LDL'')');
      | text(0.12,0.15,'[m x m]');
  P_Reshape : Reshape  OutputDimensionality=Customize  OutputDimensions=[len_state, len_state]
  P_prd Trans : Math  Operator=transpose  SaturateOnIntegerOverflow=on
  P_prd-K*H*P_prd : Sum  Inputs=-+  OutDataTypeStr=Inherit: Inherit via back propagation  InputSameDT=on
  P_prd_Reshape : Reshape  OutputDimensionality=Column vector (2-D)
  X_prd+K*(Z-H*X_prd) : Sum  InputSameDT=on  OutDataTypeStr=Inherit: Same as first input
  Z-H*X_prd : Sum  Inputs=+-  InputSameDT=on  OutDataTypeStr=Inherit: Same as first input
  Z_est_Multiply : Product  Multiplication=Matrix(*)  InputSameDT=on  OutDataTypeStr=Inherit: Same as first input
  Z_prd_Multiply : Product  Multiplication=Matrix(*)  OutDataTypeStr=Inherit: Same as first input
  Z_est : Outport
  Z_prd : Outport  Port=2
  X_prd : Outport  Port=3
  P_prd : Outport  Port=4
  wires:
  Z_prd_Multiply/1 -> Z_prd/1
  [H] -> Z_prd_Multiply/1
  A*X/1 -> Z_prd_Multiply/2, X_prd/1
  A*P*At+Q/1 -> P_prd_Reshape/1
  P_prd-K*H*P_prd/1 -> A*P*At/2
  X/1 -> X_prd+K*(Z-H*X_prd)/1, H*X_prd/2
  P/1 -> P_Reshape/1
  Z-H*X_prd/1 -> K*(Z-H*X_prd)/2
  K*(Z-H*X_prd)/1 -> X_prd+K*(Z-H*X_prd)/2
  H*X_prd/1 -> Z-H*X_prd/2
  [K] -> K*H*P_prd/1
  [H] -> K*H*P_prd/2
  K*H*P_prd/1 -> P_prd-K*H*P_prd/1
  A*P*At/1 -> A*P*At+Q/1
  Constant5/1 -> A*P*At+Q/2
  Constant4/1 -> A*P*At/3
  Constant2/1 -> H*P_prdt*Ht+R/2
  H*P_prdt*Ht/1 -> H*P_prdt*Ht+R/1
  Z/1 -> Z-H*X_prd/1
  [K] -> K*(Z-H*X_prd)/1
  [H] -> H*X_prd/1
  K Trans/1 -> [K]
  P_prd Trans/1 -> H*P_prdt/2
  H*P_prdt/1 -> LDL Solver/2(B), H*P_prdt*Ht/1
  H*P_prdt*Ht+R/1 -> LDL Solver/1(S)
  LDL Solver/1(X) -> K Trans/1
  P_prd_Reshape/1 -> P_prd/1
  [H] -> Z_est_Multiply/1
  Z_est_Multiply/1 -> Z_est/1
  X_prd+K*(Z-H*X_prd)/1 -> A*X/2, Z_est_Multiply/2
  [A] -> A*X/1
  Constant3/1 -> A*P*At/1, [A]
  P_Reshape/1 -> K*H*P_prd/3, P_prd-K*H*P_prd/2, P_prd Trans/1
  Hcst/1 -> [H], H*P_prdt/1
  Hcst_t/1 -> H*P_prdt*Ht/2

== system vipldws_fixpt/Lane Tracking/Kalman Filter (In order to change fixed-point data settings, the link to the library is disabled.)/Control/Options/P_prd_Assign ==
  In : Inport
  Ini Value : Inport  Port=2
  Assignment : Assignment  NumberOfDimensions=2  IndexOptions=Assign all,Index vector (port)  Indices=-1,1  OutputSizes=slselsubs([num_rows, num_cols],1),slselsubs([num_rows, num_cols],2)
  Reset_Value : Constant  Value=param.P  VectorParams1D=off  OutDataTypeStr=Inherit: Inherit via back propagation
  Switch : Switch  Criteria=u2 ~= 0  SaturateOnIntegerOverflow=on  InputSameDT=on
  Out : Outport
  wires:
  [Index] -> Assignment/3
  Ini Value/1 -> Assignment/1
  Assignment/1 -> Out/1
  Reset_Value/1 -> Switch/1
  [Reset] -> Switch/2
  In/1 -> Switch/3
  Switch/1 -> Assignment/2

== system vipldws_fixpt/Lane Tracking/Kalman Filter (In order to change fixed-point data settings, the link to the library is disabled.)/Control/Options/X_prd_Assign ==
  In : Inport
  Ini Value : Inport  Port=2
  Assignment : Assignment  NumberOfDimensions=2  IndexOptions=Assign all,Index vector (port)  Indices=-1,1  OutputSizes=slselsubs([num_rows, num_cols],1),slselsubs([num_rows, num_cols],2)
  Reset_Value : Constant  Value=param.X  VectorParams1D=off  OutDataTypeStr=Inherit: Inherit via back propagation
  Switch : Switch  Criteria=u2 ~= 0  SaturateOnIntegerOverflow=on  InputSameDT=on
  Out : Outport
  wires:
  Assignment/1 -> Out/1
  Ini Value/1 -> Assignment/1
  [Index] -> Assignment/3
  Reset_Value/1 -> Switch/1
  [Reset] -> Switch/2
  In/1 -> Switch/3
  Switch/1 -> Assignment/2

== system vipldws_fixpt/Lane Tracking/Kalman Filter (In order to change fixed-point data settings, the link to the library is disabled.)/Control/Options/Z_est_Assign ==
  In : Inport
  Assignment : Assignment  NumberOfDimensions=2  OutputInitialize=Specify size for each dimension in table  IndexOptions=Assign all,Index vector (port)  Indices=-1,1  OutputSizes=slselsubs([num_rows, num_cols],1),slselsubs([num_rows, num_cols],2)
  Reset_Value : Constant  Value=reset_value  VectorParams1D=off  OutDataTypeStr=Inherit: Inherit via back propagation
  Switch : Switch  Criteria=u2 ~= 0  SaturateOnIntegerOverflow=on  InputSameDT=on
  Out : Outport
  wires:
  [Index] -> Assignment/2
  Assignment/1 -> Out/1
  Reset_Value/1 -> Switch/1
  [Reset] -> Switch/2
  In/1 -> Switch/3
  Switch/1 -> Assignment/1

== system vipldws_fixpt/Lane Tracking/Matching/Calculate the distances between the lines found in the current frame and those in the repository/Select a line from the repository; if it is valid (Count > 0), Calculate its distance to the input lines./Calculate the distances between the chosen line in the repository and all input lines. ==
  note: Calculate the distance between the chosen line in the repository and every input line.
  Dis : Inport
  Rep_ref : Inport  Port=2
  Line : Inport  Port=3
  Enable : Inport  Port=4
  Assignment : Assignment  IndexOptions=Index vector (port)  Indices=1  OutputSizes=[1 1]
  Constant : Constant  Value=intmax('int16')  VectorParams1D=off  OutDataTypeStr=int32
  Difference between two lines : Subsystem
  For Iterator : ForIterator  ResetStates=reset  IterationLimit=expLaneNum
  Selector1 : Selector  NumberOfDimensions=2  InputPortWidth=3  IndexOptions=Select all,Index vector (port)  Indices=-1,-1  OutputSizes=1
  Selector2 : Selector  NumberOfDimensions=2  InputPortWidth=3  IndexOptions=Select all,Index vector (port)  Indices=-1,-1  OutputSizes=1
  Switch1 : Switch  Criteria=u2 ~= 0
  Dis_out : Outport
  wires:
  Switch1/1 -> Assignment/2
  Assignment/1 -> Dis_out/1
  Dis/1 -> Assignment/1
  Rep_ref/1 -> Difference between two lines/1(Line_1)
  For Iterator/1 -> Assignment/3, Selector2/2, Selector1/2
  Line/1 -> Selector1/1
  Enable/1 -> Selector2/1
  Selector2/1 -> Difference between two lines/Enable, Switch1/2
  Difference between two lines/1(Dis) -> Switch1/1
  Constant/1 -> Switch1/3
  Selector1/1 -> Difference between two lines/2(Line_2)

== system vipldws_fixpt/Lane Tracking/Kalman Filter (In order to change fixed-point data settings, the link to the library is disabled.)/Control/Options/Core/LDL Solver ==
  S : Inport
  B : Inport  Port=2
  Backward Substitution : dspsolvers/Backward Substitution  Unit=on  RealDiag=on  outputMin=[]  outputMax=[]  accumDataTypeStr=Inherit: Same as product output  accumLastDataTypeStr=Inherit: Same as product output  roundingMode=Floor  overflowMode=off
  Extract Diagonal : dspmtrx3/Extract Diagonal
  Forward Substitution : dspsolvers/Forward Substitution  Unit=on  RealDiag=on  outputMin=[]  outputMax=[]  accumDataTypeStr=Inherit: Same as product output  accumLastDataTypeStr=Inherit: Same as product output  roundingMode=Floor  overflowMode=off
  LDL Factorization : dspfactors/LDL Factorization  errmode=Warning  outputMin=[]  outputMax=[]  roundingMode=Floor  overflowMode=off
  Math Function : Math  Operator=reciprocal  SaturateOnIntegerOverflow=on
  Matrix Scaling : dspmtrx3/Array-Vector Multiply  mode=Mute  saveAsFlag=0  Dimension=1  V_Source=Input port  V_VectFromMask=[0.5 0.25]  firstCoeffSignedness=Auto  firstCoeffDataTypeStr=Inherit: Same word length as input  firstCoeffLastDataTypeStr=Inherit: Same word length as input  firstCoeffMin=[]  firstCoeffMax=[]  outputSignedness=Auto  outputDataTypeStr=Inherit: Same as product output  outputLastDataTypeStr=Inherit: Same as product output  outputMin=[]  outputMax=[]  accumSignedness=Auto  prodOutputSignedness=Auto  roundingMode=Floor  overflowMode=off
  X : Outport  InitialOutput=0
  wires:
  Math Function/1 -> Matrix Scaling/2
  Extract Diagonal/1 -> Math Function/1  "d"
  Matrix Scaling/1 -> Backward Substitution/2
  Forward Substitution/1 -> Matrix Scaling/1  "y"
  S/1 -> LDL Factorization/1
  B/1 -> Forward Substitution/2
  LDL Factorization/1 -> Extract Diagonal/1, Forward Substitution/1, Backward Substitution/1
  Backward Substitution/1 -> X/1

== system vipldws_fixpt/Lane Tracking/Matching/Calculate the distances between the lines found in the current frame and those in the repository/Select a line from the repository; if it is valid (Count > 0), Calculate its distance to the input lines./Calculate the distances between the chosen line in the repository and all input lines./Difference between two lines ==
  note: Distance between two lines equals to
      | abs( Rho1 - Rho2) + abs( Theta1 - Theta2) * estImageSize,
      | where estImageSize is the estimated size of the image.
  Line_1 : Inport
  Line_2 : Inport  Port=2
  Enable : EnablePort  PropagateVarSize=During execution
  Abs : Abs
  Abs1 : Abs
  Add1 : Sum  Inputs=+-  OutDataTypeStr=int32
  Add7 : Sum  OutDataTypeStr=Inherit: Same as first input
  Add8 : Sum  Inputs=+-
  Constant : Constant
  Constant1 : Constant  Value=2
  Gain : Gain  Gain=distanceMetricWeight  OutDataTypeStr=Inherit: Inherit via back propagation
  Rho_1 : Selector  InputPortWidth=2  IndexOptions=Index vector (dialog)  Indices=1  OutputSizes=1
  Rho_2 : Selector  InputPortWidth=2  IndexOptions=Index vector (port)  Indices=1  OutputSizes=1
  Theta_1 : Selector  InputPortWidth=2  IndexOptions=Index vector (dialog)  Indices=2  OutputSizes=1
  Theta_2 : Selector  InputPortWidth=2  IndexOptions=Index vector (port)  Indices=2  OutputSizes=1
  Dis : Outport
  wires:
  Gain/1 -> Add7/2
  Abs1/1 -> Add7/1
  Rho_2/1 -> Add1/2
  Rho_1/1 -> Add1/1
  Add1/1 -> Abs1/1
  Abs/1 -> Gain/1
  Add7/1 -> Dis/1
  Add8/1 -> Abs/1
  Theta_2/1 -> Add8/2
  Theta_1/1 -> Add8/1
  Line_2/1 -> Rho_2/1, Theta_2/1
  Line_1/1 -> Theta_1/1, Rho_1/1
  Constant/1 -> Rho_2/2
  Constant1/1 -> Theta_2/2

== matlab function vipldws_fixpt/Output/Exclude 3rd Lane ==
  data: in3rdLane input; out3rdLane output; Show3rdLane input; mainTwoLanes input; twoLanesFlag input; RefImg input
function out3rdLane =Exclude3rdLane(in3rdLane, Show3rdLane, mainTwoLanes, twoLanesFlag, RefImg)  

% Exclude third (left or right lane) if it is very close to the other lane 
% already detected and tracked by Kalman filter.

rH = int32(size(RefImg(:,:,1), 1));
cW = int32(size(RefImg(:,:,1), 2));

zeroI32 = int32(0);

out3rdLane = in3rdLane;  

if (Show3rdLane && twoLanesFlag)
    R1C1R2C2 = in3rdLane;
    R1 = R1C1R2C2(1)+int32(1); 
    C1 = R1C1R2C2(2)+int32(1); 
    R2 = R1C1R2C2(3)+int32(1);  
    C2 = R1C1R2C2(4)+int32(1);  
    % make sure R1 is the min(R1,R2)
    if R1>R2
        TMP=R2;
        R2=R1;
        R1=TMP;

        TMP=C2;
        C2=C1;
        C1=TMP;   
    end
    
  for lineIdx =int32(1):int32(2)  
    
    r1c1r2c2 = mainTwoLanes(:,lineIdx);
    r1 = r1c1r2c2(1)+int32(1);  
    c1 = r1c1r2c2(2)+int32(1);  
    r2 = r1c1r2c2(3)+int32(1);  
    c2 = r1c1r2c2(4)+int32(1); 

    % make sure r1 is the min(r1,r2)
    if r1>r2
        tmp=r2;
        r2=r1;
        r1=tmp;

        tmp=c2;
        c2=c1;
        c1=tmp;   
    end
    
    pointNotLine = (r1==r2) && (c1==c2);
    
    % find if line is within image: (r1,c1)  and (r2,c2) must be within image
    if ((r1>zeroI32 && r1 <= rH) && (c1>zeroI32 && c1 <= cW) && ...
        (r2>zeroI32 && r2 <= rH) && (c2>zeroI32 && c2 <= cW)) && ~pointNotLine
        %line_within_image = true;
        if (abs(r1-R1)+ abs(c1-C1) + abs(r2-R2) +abs(c2-C2))< int32(20)
            out3rdLane = int32([-1000 -1000 -1000 -1000]');
        end            
    else
       % line outside image
       % go to nextLine
    end    
  end    
else
   out3rdLane = in3rdLane;  
end

== matlab function vipldws_fixpt/Departure Warning/Departure detection/subsystem/Combine Left Right Departure ==
  data: curMsg input; prevMsg input int8; outMsg output; numNormalDrivenFrames input
function outMsg=CombineLeftRightDeparture(curMsg, prevMsg, numNormalDrivenFrames)  

% It combines left-right departure to left departure
%         and right-left departure to right departure
% It utilizes the fact that there must be at least 4 frames of normal driving 
% between a left departure warning and a right departure warning

%RIGHT_DEP=0; NORMAL=1; LEFT_DEP=2
NORMAL = int8(1);

if curMsg == NORMAL
    outMsg = NORMAL;
else % curMsg == RIGHT_DEP  || curMsg == LEFT_DEP
    if (numNormalDrivenFrames < int32(4))
        % use the previous message
        outMsg = prevMsg;        
    else
        outMsg = curMsg;
    end        
end
